simulink model "MBC11_IPC_twr_accel"  (R2017b)
settings: Solver=ode45  StartTime=0.0  StopTime=TMax  RelTol=1e-3  EnableMultiTasking=on
values from neighbouring files (symbols this model uses):
  alpha = exp(-2*pi*DT*fc)    [MBC_11_IPC.m]    (also in MBC_11_IPC_twr_accel.m)
  Dbar = zeros(size(Gbar,1),size(Kbar',2))    [MBC_11_IPC.m]    (also in MBC_11_IPC_twr_accel.m)
  DT = 0.01    [MBC_11_IPC.m]    (also in MBC_11_IPC_twr_accel.m)
  Gbar = [G 4*Gd]    [MBC_11_IPC.m]    (also in MBC_11_IPC_twr_accel.m)
  Lbar = (Abar + Bbar*Gbar - Kbar'*Cbar)    [MBC_11_IPC.m]    (also in MBC_11_IPC_twr_accel.m)
  PC_MaxPit = 1.570796    [MBC_11_IPC.m]    (also in MBC_11_IPC_twr_accel.m)
  PC_MaxRat = 0.1396263    [MBC_11_IPC.m]    (also in MBC_11_IPC_twr_accel.m)
  PC_MinPit = 0.0    (= 0)    [MBC_11_IPC.m]    (also in MBC_11_IPC_twr_accel.m)
  ref_pitch = 7.13132E-02    (= 0.0713132)    [MBC_11_IPC.m]    (also in MBC_11_IPC_twr_accel.m)
  ref_rot = 1.266999999999998    (= 1.267)    [MBC_11_IPC.m]    (also in MBC_11_IPC_twr_accel.m)
undefined symbols (not defined in the file or in its folder): OutList, strmatch
settings Model: Creator=Avell 1513  LastModifiedBy=Avell 1513
settings DataIOCC: LimitDataPoints=on  SaveFormat=Array
settings OptimizationCC: LifeSpan=inf
settings DebuggingCC: UnderspecifiedInitializationDetection=Classic  MergeDetectMultiDrivingBlocksExec=none  SolverPrmCheckMsg=warning  StateNameClashWarn=warning  SFUnexpectedBacktrackingDiag=warning  SFNoUnconditionalDefaultTransitionDiag=warning  SFExecutionAtInitializationDiag=none
settings HardwareCC: ProdBitPerPointer=32  ProdBitPerSizeT=32  ProdBitPerPtrDiffT=32  ProdLargestAtomicFloat=None  ProdIntDivRoundTo=Undefined  ProdEndianess=Unspecified  ProdWordSize=32  ProdHWDeviceType=32-bit Generic
settings ModelReferenceCC: PropagateSignalLabelsOutOfModel=off
settings CodeAppCC: StateflowObjectComments=on
settings GRTTargetCC: TargetLangStandard=C89/C90 (ANSI)  GeneratePreprocessorConditionals=Disable all
settings ConfigComp: CovMetricSettings=dw  CovHtmlReporting=on  CovSaveCumulativeToWorkspaceVar=on  CovSaveSingleToWorkspaceVar=on  CovExternalEMLEnable=off

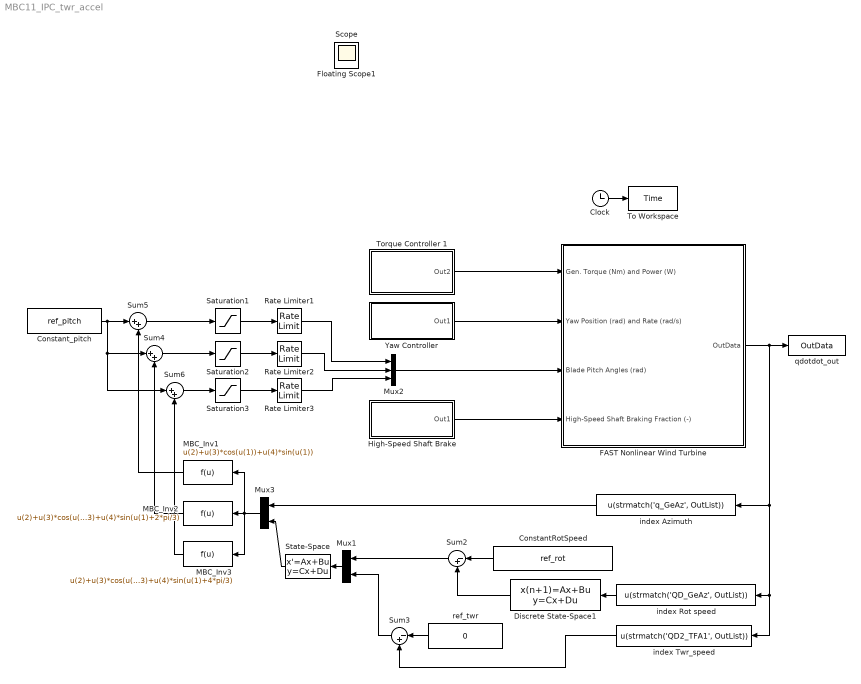
== system MBC11_IPC_twr_accel ==
  Clock : Clock
  ConstantRotSpeed : Constant  Value=ref_rot
  Constant_pitch : Constant  Value=ref_pitch
  Discrete State-Space1 : DiscreteStateSpace  A=alpha  B=1-alpha  C=alpha  D=1-alpha  InitialCondition=ref_rot  SampleTime=DT
  FAST Nonlinear Wind Turbine : Subsystem  mask(FAST Nonlinear Wind Turbine){}
      mask help: This block contains the FAST S-Function.
      mask init:
      | clear FAST_SFunc
  High-Speed Shaft Brake : Subsystem
  MBC_Inv1 : Fcn  Expr=u(2)+u(3)*cos(u(1))+u(4)*sin(u(1))
  MBC_Inv2 : Fcn  Expr=u(2)+u(3)*cos(u(1)+2*pi/3)+u(4)*sin(u(1)+2*pi/3)
  MBC_Inv3 : Fcn  Expr=u(2)+u(3)*cos(u(1)+4*pi/3)+u(4)*sin(u(1)+4*pi/3)
  Mux1 : Mux  Inputs=2
  Mux2 : Mux  Inputs=3
  Mux3 : Mux  Inputs=2
  Rate Limiter1 : RateLimiter  RisingSlewLimit=PC_MaxRat  FallingSlewLimit=-PC_MaxRat  SampleTimeMode=inherited  LinearizeAsGain=off
  Rate Limiter2 : RateLimiter  RisingSlewLimit=PC_MaxRat  FallingSlewLimit=-PC_MaxRat  SampleTimeMode=inherited  LinearizeAsGain=off
  Rate Limiter3 : RateLimiter  RisingSlewLimit=PC_MaxRat  FallingSlewLimit=-PC_MaxRat  SampleTimeMode=inherited  LinearizeAsGain=off
  Saturation1 : Saturate  UpperLimit=PC_MaxPit  LowerLimit=PC_MinPit
  Saturation2 : Saturate  UpperLimit=PC_MaxPit  LowerLimit=PC_MinPit
  Saturation3 : Saturate  UpperLimit=PC_MaxPit  LowerLimit=PC_MinPit
  State-Space : StateSpace  A=Lbar  B=Kbar'  C=Gbar  D=Dbar  InitialCondition=0
  Sum2 : Sum  Inputs=|-+
  Sum3 : Sum  Inputs=|-+
  Sum4 : Sum  Inputs=|++
  Sum5 : Sum  Inputs=|++
  Sum6 : Sum  Inputs=|++
  To Workspace : ToWorkspace  VariableName=Time  SampleTime=-1
  Torque Controller 1 : Subsystem
  Yaw Controller : Subsystem
  index Azimuth : Fcn  Expr=u(strmatch('q_GeAz', OutList))
  index Rot speed : Fcn  Expr=u(strmatch('QD_GeAz', OutList))
  index Twr_speed : Fcn  Expr=u(strmatch('QD2_TFA1', OutList))
  qdotdot_out : ToWorkspace  VariableName=OutData  SampleTime=-1
  ref_twr : Constant  Value=0
  Floating Scope1 : Scope
  Scope : Scope
  wires:
  Yaw Controller/1(Out1) -> FAST Nonlinear Wind Turbine/2(Yaw Position (rad) and Rate (rad/s))
  High-Speed Shaft Brake/1(Out1) -> FAST Nonlinear Wind Turbine/4(High-Speed Shaft Braking Fraction (-))
  Clock/1 -> To Workspace/1
  FAST Nonlinear Wind Turbine/1(OutData) -> index Rot speed/1, index Twr_speed/1, index Azimuth/1, qdotdot_out/1
  Torque Controller 1/1(Out2) -> FAST Nonlinear Wind Turbine/1(Gen. Torque (Nm) and Power (W))
  ConstantRotSpeed/1 -> Sum2/1
  index Twr_speed/1 -> Sum3/2
  Mux1/1 -> State-Space/1
  ref_twr/1 -> Sum3/1
  Discrete State-Space1/1 -> Sum2/2
  index Rot speed/1 -> Discrete State-Space1/1
  Sum3/1 -> Mux1/2
  Sum2/1 -> Mux1/1
  Sum6/1 -> Saturation3/1
  Sum4/1 -> Saturation2/1
  Rate Limiter2/1 -> Mux2/2
  MBC_Inv1/1 -> Sum5/2
  Rate Limiter1/1 -> Mux2/1
  Constant_pitch/1 -> Sum6/1, Sum4/1, Sum5/1
  MBC_Inv3/1 -> Sum6/2
  Rate Limiter3/1 -> Mux2/3
  Saturation1/1 -> Rate Limiter1/1
  Saturation3/1 -> Rate Limiter3/1
  Saturation2/1 -> Rate Limiter2/1
  Sum5/1 -> Saturation1/1
  MBC_Inv2/1 -> Sum4/2
  Mux2/1 -> FAST Nonlinear Wind Turbine/3(Blade Pitch Angles (rad))
  index Azimuth/1 -> Mux3/1
  State-Space/1 -> Mux3/2
  Mux3/1 -> MBC_Inv3/1, MBC_Inv1/1, MBC_Inv2/1

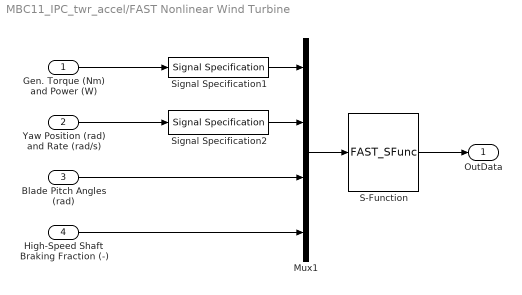
== system MBC11_IPC_twr_accel/FAST Nonlinear Wind Turbine ==
  Gen. Torque (Nm) and Power (W) : Inport
  Yaw Position (rad) and Rate (rad/s) : Inport  Port=2
  Blade Pitch Angles (rad) : Inport  Port=3
  High-Speed Shaft Braking Fraction (-) : Inport  Port=4
  Mux1 : Mux
  S-Function : S-Function  FunctionName=FAST_SFunc  Parameters=FAST_InputFileName, TMax, 0  SFunctionDeploymentMode=off  EnableBusSupport=off
  Signal Specification1 : SignalSpecification  OutDataTypeStr=double  Dimensions=2
  Signal Specification2 : SignalSpecification  OutDataTypeStr=double  Dimensions=2
  OutData : Outport
  wires:
  Gen. Torque (Nm) and Power (W)/1 -> Signal Specification1/1
  S-Function/1 -> OutData/1
  Mux1/1 -> S-Function/1
  Blade Pitch Angles (rad)/1 -> Mux1/3
  Yaw Position (rad) and Rate (rad/s)/1 -> Signal Specification2/1
  Signal Specification1/1 -> Mux1/1
  Signal Specification2/1 -> Mux1/2
  High-Speed Shaft Braking Fraction (-)/1 -> Mux1/4

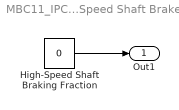
== system MBC11_IPC_twr_accel/High-Speed Shaft Brake ==
  High-Speed Shaft Braking Fraction : Constant  Value=0
  Out1 : Outport
  wires:
  High-Speed Shaft Braking Fraction/1 -> Out1/1

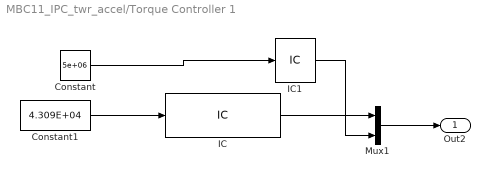
== system MBC11_IPC_twr_accel/Torque Controller 1 ==
  Constant : Constant  Value=5e+06
  Constant1 : Constant  Value=4.309E+04
  IC : InitialCondition  Value=4.309E+04
  IC1 : InitialCondition  Value=5e+06
  Mux1 : Mux  Inputs=2
  Out2 : Outport
  wires:
  Mux1/1 -> Out2/1
  IC/1 -> Mux1/1
  IC1/1 -> Mux1/2
  Constant/1 -> IC1/1
  Constant1/1 -> IC/1

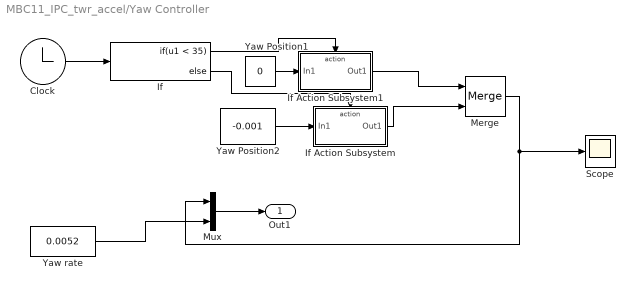
== system MBC11_IPC_twr_accel/Yaw Controller ==
  Clock : Clock
  If : If  IfExpression=u1 < 35
  If Action Subsystem : Subsystem  TreatAsAtomicUnit=on
  If Action Subsystem1 : Subsystem  TreatAsAtomicUnit=on
  Merge : Merge
  Mux : Mux  Inputs=2
  Scope : Scope
  Yaw Position1 : Constant  Value=0
  Yaw Position2 : Constant  Value=-0.001
  Yaw rate : Constant  Value=0.0052
  Out1 : Outport
  wires:
  Mux/1 -> Out1/1
  Yaw rate/1 -> Mux/2
  If Action Subsystem/1(Out1) -> Merge/2
  Clock/1 -> If/1
  If/1 -> If Action Subsystem1/Action
  Yaw Position1/1 -> If Action Subsystem1/1(In1)
  If/2 -> If Action Subsystem/Action
  Yaw Position2/1 -> If Action Subsystem/1(In1)
  If Action Subsystem1/1(Out1) -> Merge/1
  Merge/1 -> Scope/1, Mux/1

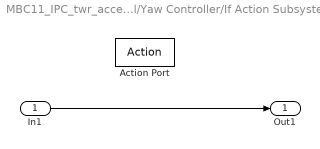
== system MBC11_IPC_twr_accel/Yaw Controller/If Action Subsystem ==
  In1 : Inport
  Action Port : ActionPort  ActionType=else
  Out1 : Outport
  wires:
  In1/1 -> Out1/1

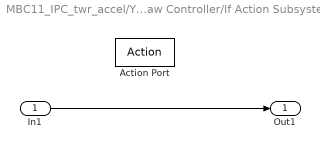
== system MBC11_IPC_twr_accel/Yaw Controller/If Action Subsystem1 ==
  In1 : Inport
  Action Port : ActionPort  ActionType=then
  Out1 : Outport
  wires:
  In1/1 -> Out1/1
